simulink model "Passive_balancing"  (R2021b)
settings: Solver=VariableStepAuto  StartTime=0.0  StopTime=10.0  RelTol=1e-3
values from neighbouring files (symbols this model uses):
  I_cc = 4    [Passive_balancing.m]
  I_gain = 10    [Passive_balancing.m]
  P_gain = 100    [Passive_balancing.m]
  R_bleed = 20    [Passive_balancing.m]
  T_volt = 600    [Passive_balancing.m]
  V_top = 4.1    [Passive_balancing.m]
undefined symbols (not defined in the file or in its folder): Battery
libraries: fl_lib x36, nesl_utility x23, ee_lib x8, simulink x3, slpidlib x1
settings Model: Creator=vijay  LastModifiedBy=vijay

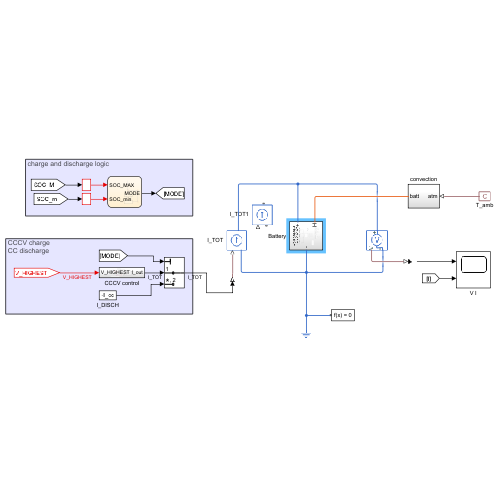
[thumbnail: Simulink's stored preview of the top-level diagram]
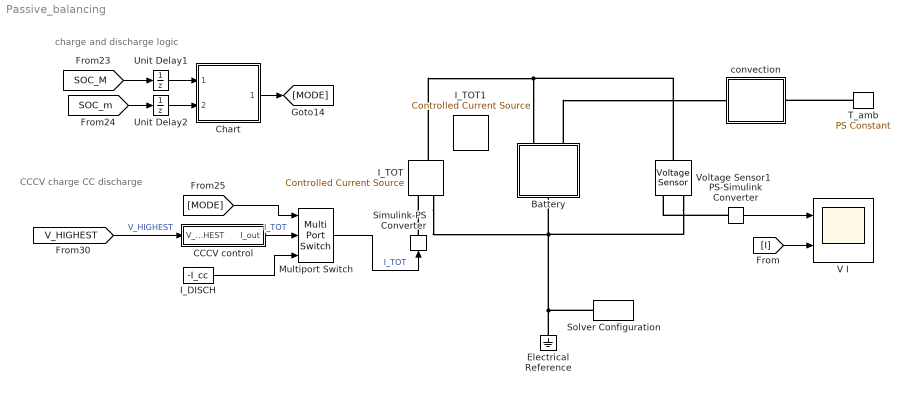
== system Passive_balancing ==
  note: charge and discharge logic
  note: CCCV charge
      | CC discharge
  Battery : Subsystem
  CCCV control : Subsystem
  Chart : Stateflow chart  TreatAsAtomicUnit=on
  Electrical Reference : fl_lib/Electrical/Electrical Elements/Electrical Reference
  I_DISCH : Constant  Value=-I_cc
  I_TOT : fl_lib/Electrical/Electrical Sources/Controlled Current Source
  I_TOT1 : fl_lib/Electrical/Electrical Sources/Controlled Current Source
  Multiport Switch : MultiPortSwitch  DataPortOrder=Specify indices  DataPortIndices={1,2}  DiagnosticForDefault=None
  PS-Simulink Converter : nesl_utility/PS-Simulink Converter  PhysicalDomain=network_engine_domain  SubClassName=ps_output  LeftPortType=input  RightPortType=output  PseudoPeriodic=off  Frequencies=[]  Unit=inherit  AffineConversion=off
      settings: SourceProductBaseCode=PW,SS
  Simulink-PS Converter : nesl_utility/Simulink-PS Converter  PhysicalDomain=network_engine_domain  SubClassName=ps_input  LeftPortType=input  RightPortType=output  PseudoPeriodic=off  Frequencies=[]  NoiseDistribution=none  NoiseParameters=[]  Unit=1  AffineConversion=off  FilteringAndDerivatives=provide  SimscapeFilterOrder=1  InputFilterTimeConstant=0.001  UdotUserProvided=0
      settings: SourceProductBaseCode=PW,SS
  Solver Configuration : nesl_utility/Solver Configuration  PhysicalDomain=network_engine_domain  SubClassName=solver  LeftPortType=input  RightPortType=generic  Tones=[]  Harmonics=[]  SimulateNoise=off  Profile=off  UseLocalSampling=off  EnableSwitchedLinearOptims=on  FrequencyDomain=off  UseCCode=off  RelTol=0.001  AbsTol=1e-06  MinStep=1e-09  ToWorkspace=off  RevertToSquareIcSolve=off  NumHomotopyIterations=100  PhasorMode=off  PhasorModeNumHarmonics=1  DoDC=off  ResidualTolerance=1e-09  UseLocalSolver=on  LocalSolverChoice=NE_BACKWARD_EULER_ADVANCER  LocalSolverSampleTime=1  DoFixedCost=on  MaxNonlinIter=3  MaxModeIter=2  ComputeImpulses=off  ImpulseIterations=2  LinearAlgebra=Sparse  EquationFormulation=NE_TIME_EF  DelaysMemoryBudget=1024  AutomaticFiltering=on  FilteringTimeConstant=0.001  PartitionStorageMethod=AS_NEEDED  PartitionMemoryBudget=1024  PartitionMethod=FAST
      settings: SourceProductBaseCode=PW,SS
  T_amb : fl_lib/Physical Signals/Sources/PS Constant  constant=20+273
  Unit Delay1 : UnitDelay  InitialCondition=1  SampleTime=-1  HasFrameUpgradeWarning=on
  Unit Delay2 : UnitDelay  InitialCondition=1  SampleTime=-1  HasFrameUpgradeWarning=on
  V I : Scope  NumInputPorts=2
  Voltage Sensor1 : fl_lib/Electrical/Electrical Sensors/Voltage Sensor
  convection : Subsystem
  wires:
  PS-Simulink Converter/1 -> V I/1
  [I] -> V I/2
  [V_HIGHEST] -> CCCV control/1(V_HIGHEST)  "V_HIGHEST"
  Unit Delay1/1 -> Chart/1(SOC_MAX)
  [SOC_M] -> Unit Delay1/1
  Unit Delay2/1 -> Chart/2(SOC_min)
  Chart/1(MODE) -> [MODE]
  I_DISCH/1 -> Multiport Switch/3
  CCCV control/1(I_out) -> Multiport Switch/2  "I_TOT"
  [SOC_m] -> Unit Delay2/1
  [MODE] -> Multiport Switch/1
  Multiport Switch/1 -> Simulink-PS Converter/1  "I_TOT"
  connections:
  Voltage Sensor1/LConn1 -- I_TOT/LConn1 -- Battery/LConn1
  Battery/LConn2 -- convection/LConn1
  Solver Configuration/RConn1 -- Voltage Sensor1/RConn2 -- I_TOT/RConn2 -- Battery/RConn1 -- Electrical Reference/LConn1
  T_amb/RConn1 -- convection/RConn1
  PS-Simulink Converter/LConn1 -- Voltage Sensor1/RConn1
  Simulink-PS Converter/RConn1 -- I_TOT/RConn1

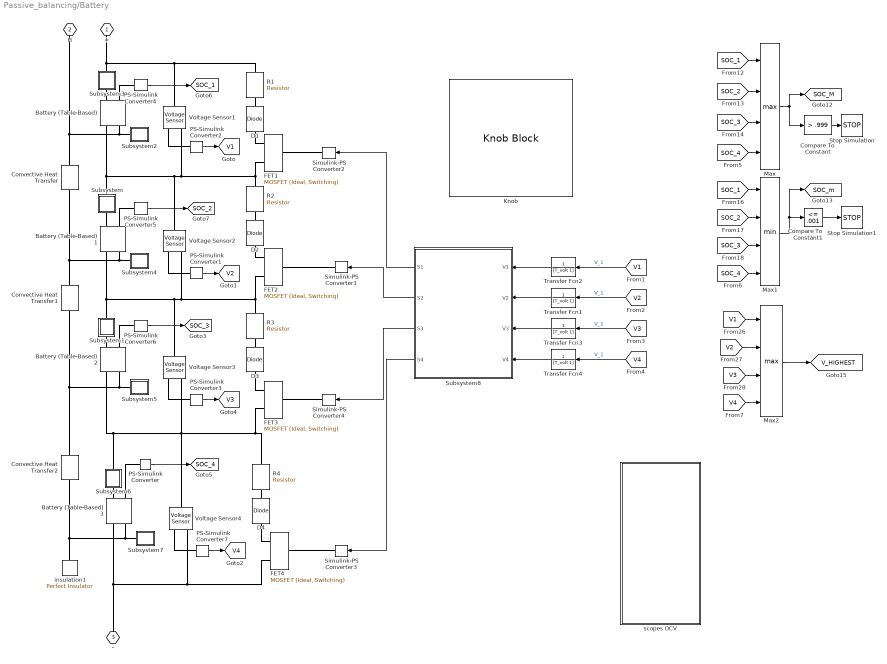
== system Passive_balancing/Battery ==
  Battery (Table-Based) : ee_lib/Sources/Battery (Table-Based)  SOC_vec=Battery(1).SOC_LUT  T_dependence=ee.enum.temperature_dependence.yes  prm_dir=ee.enum.battery.prm_dir.noCurrentDirectionality  T_vec=Battery(1).Temperature_LUT K  V0_mat=Battery(1).Em_LUT V  V0_vec=[3.1, 3.27, 3.31, 3.5] V  R0_mat=Battery(1).R0_LUT Ohm  R0_vec=[.015, .017, .012, .013] Ohm  R0_dis_mat=[.03, .015, .002; .04, .017, .008; .039, .012, .006; .027, .013, .021] Ohm  R0_dis_vec=[.015, .017, .012, .013] Ohm  R0_ch_mat=[.03, .015, .002; .04, .017, .008; .039, .012, .006; .027, .013, .021] Ohm  R0_ch_vec=[.015, .017, .012, .013] Ohm  AH_vec=Battery(1).Capacity_LUT A*hr  AH=4.1 A*hr  prm_leak=ee.enum.battery.prm_leak.disabled  Rleak_vec=[8000, 7000, 6000] Ohm  Rleak=7e3 Ohm  extrapolation_option=ee.enum.extrapolation.linear  prm_dyn=ee.enum.battery.prm_dyn.rc3  R1_mat=Battery(1).R1_LUT Ohm  R1_vec=[.076, .022, .007, .043] Ohm  tau1_mat=Battery(1).t1_LUT s  tau1_vec=[148, 110, 27, 22] s  R2_mat=Battery(1).R2_LUT Ohm  R2_vec=[.382, .006, .007, .956] Ohm  tau2_mat=Battery(1).t2_LUT s  tau2_vec=[44, 24, 14, 13419] s  R3_mat=Battery(1).R3_LUT Ohm  R3_vec=[.382, .006, .007, .956] Ohm  tau3_mat=Battery(1).t3_LUT s  tau3_vec=[44, 24, 14, 13419] s  R4_mat=Battery(1).R4_LUT Ohm  R4_vec=[.382, .006, .007, .956] Ohm  tau4_mat=Battery(1).t4_LUT s  tau4_vec=[44, 24, 14, 13419] s  R5_mat=[.014, .382, .407; .028, .006, .007; .014, .007, .006; .333, .956, .912] Ohm  R5_vec=[.382, .006, .007, .956] Ohm  tau5_mat=[1, 44, 5644; 11, 24, 506; 2, 14, 330; 3310, 13419, 30216] s  tau5_vec=[44, 24, 14, 13419] s  prm_fade=ee.enum.battery.prm_fade.equations  N0=100  dV0=0  dR0=0  dAH=0  dRleak=0  dR1=0  dR2=0  dR3=0  dR4=0  dR5=0  N0vec=[100, 200, 300]  Tfadevec=[298.15, 323.15] K  dV0vec=[0, 0, 0]  dR0vec=[0, 0, 0]  dAHvec=[0, 0, 0]  dRleakvec=[0, 0, 0]  dR1vec=[0, 0, 0]  dR2vec=[0, 0, 0]  dR3vec=[0, 0, 0]  dR4vec=[0, 0, 0]  dR5vec=[0, 0, 0]  dV0mat=[0, 0; 0, 0; 0, 0]  dR0mat=[0, 0; 0, 0; 0, 0]  dAHmat=[0, 0; 0, 0; 0, 0]  dRleakmat=[0, 0; 0, 0; 0, 0]  dR1mat=[0, 0; 0, 0; 0, 0]  dR2mat=[0, 0; 0, 0; 0, 0]  dR3mat=[0, 0; 0, 0; 0, 0]  dR4mat=[0, 0; 0, 0; 0, 0]  dR5mat=[0, 0; 0, 0; 0, 0]  prm_age=ee.enum.battery.prm_age.disabled  prm_age_OCV=ee.enum.battery.prm_age_OCV.OCV  OCV_age=0.9  SOC_age=0.6  storage_dt_age_vec=[0] d  storage_T_age_vec=[273] K  OCV_scaling_age=2.2134e6  OCV_offset_age=1.632e6  temp_exp_age=0.515833569 V  t_exp_age=0.75  T_age_vec=[273.15, 298.15, 323.15] K  dt_age_vec=[90, 180, 270, 360] d  dR0_age_vec=[0, 0, 0]  t_meas_dR0_age=100 d  dR0_age_mat=[0, 0, 0; 0, 0, 0; 0, 0, 0; 0, 0, 0]  temperature=Battery(1).T_init K  i_specify=off  i_priority=None  i=0 A  i_nominal_specify=off  i_nominal_unit=A  i_nominal_value=1  v_specify=off  v_priority=None  v=0 V  v_nominal_specify=off  v_nominal_unit=V  v_nominal_value=1  stateOfCharge_specify=on  stateOfCharge_priority=High  stateOfCharge=Battery(1).SOC0  stateOfCharge_nominal_specify=off  stateOfCharge_nominal_unit=1  stateOfCharge_nominal_value=1  num_cycles_specify=off  num_cycles_priority=High  num_cycles=0  num_cycles_nominal_specify=off  num_cycles_nominal_unit=1  num_cycles_nominal_value=1  thermal_mass=Battery(1).cell_Cp_heat * Battery(1).cell_mass J/K  temperature_specify=on  temperature_priority=High  temperature_nominal_specify=off  temperature_nominal_unit=K  temperature_nominal_value=1
      settings: SourceProductBaseCode=PS  InternalSimscapePortConfiguration="{\"Bottom\":[],\"Left\":[{\"id\":\"p\",\"label\":\"+\",\"type\":\"foundation.electrical.electrical\"},{\"id\":\"soc\",\"label\":\"SOC\",\"type\":\"output\"}],\"Right\":[{\"id\":\"n\",\"label\":\"-\",\"type\":\"foundation.electrical.electrical\"},{\"id\":\"H\",\"label\":\"H\",\"type\":\"foundation.thermal.thermal\"}],\"Top\":[]}"
  Battery (Table-Based)1 : ee_lib/Sources/Battery (Table-Based)  SOC_vec=Battery(2).SOC_LUT  T_dependence=ee.enum.temperature_dependence.yes  prm_dir=ee.enum.battery.prm_dir.noCurrentDirectionality  T_vec=Battery(2).Temperature_LUT K  V0_mat=Battery(2).Em_LUT V  V0_vec=[3.1, 3.27, 3.31, 3.5] V  R0_mat=Battery(2).R0_LUT Ohm  R0_vec=[.015, .017, .012, .013] Ohm  R0_dis_mat=[.03, .015, .002; .04, .017, .008; .039, .012, .006; .027, .013, .021] Ohm  R0_dis_vec=[.015, .017, .012, .013] Ohm  R0_ch_mat=[.03, .015, .002; .04, .017, .008; .039, .012, .006; .027, .013, .021] Ohm  R0_ch_vec=[.015, .017, .012, .013] Ohm  AH_vec=Battery(2).Capacity_LUT A*hr  AH=4.1 A*hr  prm_leak=ee.enum.battery.prm_leak.disabled  Rleak_vec=[8000, 7000, 6000] Ohm  Rleak=7e3 Ohm  extrapolation_option=ee.enum.extrapolation.linear  prm_dyn=ee.enum.battery.prm_dyn.rc3  R1_mat=Battery(2).R1_LUT Ohm  R1_vec=[.076, .022, .007, .043] Ohm  tau1_mat=Battery(2).t1_LUT s  tau1_vec=[148, 110, 27, 22] s  R2_mat=Battery(2).R2_LUT Ohm  R2_vec=[.382, .006, .007, .956] Ohm  tau2_mat=Battery(2).t2_LUT s  tau2_vec=[44, 24, 14, 13419] s  R3_mat=Battery(2).R3_LUT Ohm  R3_vec=[.382, .006, .007, .956] Ohm  tau3_mat=Battery(2).t3_LUT s  tau3_vec=[44, 24, 14, 13419] s  R4_mat=Battery(2).R4_LUT Ohm  R4_vec=[.382, .006, .007, .956] Ohm  tau4_mat=Battery(2).t4_LUT s  tau4_vec=[44, 24, 14, 13419] s  R5_mat=[.014, .382, .407; .028, .006, .007; .014, .007, .006; .333, .956, .912] Ohm  R5_vec=[.382, .006, .007, .956] Ohm  tau5_mat=[1, 44, 5644; 11, 24, 506; 2, 14, 330; 3310, 13419, 30216] s  tau5_vec=[44, 24, 14, 13419] s  prm_fade=ee.enum.battery.prm_fade.equations  N0=100  dV0=0  dR0=0  dAH=0  dRleak=0  dR1=0  dR2=0  dR3=0  dR4=0  dR5=0  N0vec=[100, 200, 300]  Tfadevec=[298.15, 323.15] K  dV0vec=[0, 0, 0]  dR0vec=[0, 0, 0]  dAHvec=[0, 0, 0]  dRleakvec=[0, 0, 0]  dR1vec=[0, 0, 0]  dR2vec=[0, 0, 0]  dR3vec=[0, 0, 0]  dR4vec=[0, 0, 0]  dR5vec=[0, 0, 0]  dV0mat=[0, 0; 0, 0; 0, 0]  dR0mat=[0, 0; 0, 0; 0, 0]  dAHmat=[0, 0; 0, 0; 0, 0]  dRleakmat=[0, 0; 0, 0; 0, 0]  dR1mat=[0, 0; 0, 0; 0, 0]  dR2mat=[0, 0; 0, 0; 0, 0]  dR3mat=[0, 0; 0, 0; 0, 0]  dR4mat=[0, 0; 0, 0; 0, 0]  dR5mat=[0, 0; 0, 0; 0, 0]  prm_age=ee.enum.battery.prm_age.disabled  prm_age_OCV=ee.enum.battery.prm_age_OCV.OCV  OCV_age=0.9  SOC_age=0.6  storage_dt_age_vec=[0] d  storage_T_age_vec=[273] K  OCV_scaling_age=2.2134e6  OCV_offset_age=1.632e6  temp_exp_age=0.515833569 V  t_exp_age=0.75  T_age_vec=[273.15, 298.15, 323.15] K  dt_age_vec=[90, 180, 270, 360] d  dR0_age_vec=[0, 0, 0]  t_meas_dR0_age=100 d  dR0_age_mat=[0, 0, 0; 0, 0, 0; 0, 0, 0; 0, 0, 0]  temperature=Battery(2).T_init K  i_specify=off  i_priority=None  i=0 A  i_nominal_specify=off  i_nominal_unit=A  i_nominal_value=1  v_specify=off  v_priority=None  v=0 V  v_nominal_specify=off  v_nominal_unit=V  v_nominal_value=1  stateOfCharge_specify=on  stateOfCharge_priority=High  stateOfCharge=Battery(2).SOC0  stateOfCharge_nominal_specify=off  stateOfCharge_nominal_unit=1  stateOfCharge_nominal_value=1  num_cycles_specify=off  num_cycles_priority=High  num_cycles=0  num_cycles_nominal_specify=off  num_cycles_nominal_unit=1  num_cycles_nominal_value=1  thermal_mass=Battery(2).cell_Cp_heat * Battery(2).cell_mass J/K  temperature_specify=on  temperature_priority=High  temperature_nominal_specify=off  temperature_nominal_unit=K  temperature_nominal_value=1
      settings: SourceProductBaseCode=PS  InternalSimscapePortConfiguration="{\"Bottom\":[],\"Left\":[{\"id\":\"p\",\"label\":\"+\",\"type\":\"foundation.electrical.electrical\"},{\"id\":\"soc\",\"label\":\"SOC\",\"type\":\"output\"}],\"Right\":[{\"id\":\"n\",\"label\":\"-\",\"type\":\"foundation.electrical.electrical\"},{\"id\":\"H\",\"label\":\"H\",\"type\":\"foundation.thermal.thermal\"}],\"Top\":[]}"
  Battery (Table-Based)2 : ee_lib/Sources/Battery (Table-Based)  SOC_vec=Battery(3).SOC_LUT  T_dependence=ee.enum.temperature_dependence.yes  prm_dir=ee.enum.battery.prm_dir.noCurrentDirectionality  T_vec=Battery(3).Temperature_LUT K  V0_mat=Battery(3).Em_LUT V  V0_vec=[3.1, 3.27, 3.31, 3.5] V  R0_mat=Battery(3).R0_LUT Ohm  R0_vec=[.015, .017, .012, .013] Ohm  R0_dis_mat=[.03, .015, .002; .04, .017, .008; .039, .012, .006; .027, .013, .021] Ohm  R0_dis_vec=[.015, .017, .012, .013] Ohm  R0_ch_mat=[.03, .015, .002; .04, .017, .008; .039, .012, .006; .027, .013, .021] Ohm  R0_ch_vec=[.015, .017, .012, .013] Ohm  AH_vec=Battery(3).Capacity_LUT A*hr  AH=4.1 A*hr  prm_leak=ee.enum.battery.prm_leak.disabled  Rleak_vec=[8000, 7000, 6000] Ohm  Rleak=7e3 Ohm  extrapolation_option=ee.enum.extrapolation.linear  prm_dyn=ee.enum.battery.prm_dyn.rc3  R1_mat=Battery(3).R1_LUT Ohm  R1_vec=[.076, .022, .007, .043] Ohm  tau1_mat=Battery(3).t1_LUT s  tau1_vec=[148, 110, 27, 22] s  R2_mat=Battery(3).R2_LUT Ohm  R2_vec=[.382, .006, .007, .956] Ohm  tau2_mat=Battery(3).t2_LUT s  tau2_vec=[44, 24, 14, 13419] s  R3_mat=Battery(3).R3_LUT Ohm  R3_vec=[.382, .006, .007, .956] Ohm  tau3_mat=Battery(3).t3_LUT s  tau3_vec=[44, 24, 14, 13419] s  R4_mat=Battery(3).R4_LUT Ohm  R4_vec=[.382, .006, .007, .956] Ohm  tau4_mat=Battery(3).t4_LUT s  tau4_vec=[44, 24, 14, 13419] s  R5_mat=[.014, .382, .407; .028, .006, .007; .014, .007, .006; .333, .956, .912] Ohm  R5_vec=[.382, .006, .007, .956] Ohm  tau5_mat=[1, 44, 5644; 11, 24, 506; 2, 14, 330; 3310, 13419, 30216] s  tau5_vec=[44, 24, 14, 13419] s  prm_fade=ee.enum.battery.prm_fade.equations  N0=100  dV0=0  dR0=0  dAH=0  dRleak=0  dR1=0  dR2=0  dR3=0  dR4=0  dR5=0  N0vec=[100, 200, 300]  Tfadevec=[298.15, 323.15] K  dV0vec=[0, 0, 0]  dR0vec=[0, 0, 0]  dAHvec=[0, 0, 0]  dRleakvec=[0, 0, 0]  dR1vec=[0, 0, 0]  dR2vec=[0, 0, 0]  dR3vec=[0, 0, 0]  dR4vec=[0, 0, 0]  dR5vec=[0, 0, 0]  dV0mat=[0, 0; 0, 0; 0, 0]  dR0mat=[0, 0; 0, 0; 0, 0]  dAHmat=[0, 0; 0, 0; 0, 0]  dRleakmat=[0, 0; 0, 0; 0, 0]  dR1mat=[0, 0; 0, 0; 0, 0]  dR2mat=[0, 0; 0, 0; 0, 0]  dR3mat=[0, 0; 0, 0; 0, 0]  dR4mat=[0, 0; 0, 0; 0, 0]  dR5mat=[0, 0; 0, 0; 0, 0]  prm_age=ee.enum.battery.prm_age.disabled  prm_age_OCV=ee.enum.battery.prm_age_OCV.OCV  OCV_age=0.9  SOC_age=0.6  storage_dt_age_vec=[0] d  storage_T_age_vec=[273] K  OCV_scaling_age=2.2134e6  OCV_offset_age=1.632e6  temp_exp_age=0.515833569 V  t_exp_age=0.75  T_age_vec=[273.15, 298.15, 323.15] K  dt_age_vec=[90, 180, 270, 360] d  dR0_age_vec=[0, 0, 0]  t_meas_dR0_age=100 d  dR0_age_mat=[0, 0, 0; 0, 0, 0; 0, 0, 0; 0, 0, 0]  temperature=Battery(3).T_init K  i_specify=off  i_priority=None  i=0 A  i_nominal_specify=off  i_nominal_unit=A  i_nominal_value=1  v_specify=off  v_priority=None  v=0 V  v_nominal_specify=off  v_nominal_unit=V  v_nominal_value=1  stateOfCharge_specify=on  stateOfCharge_priority=High  stateOfCharge=Battery(3).SOC0  stateOfCharge_nominal_specify=off  stateOfCharge_nominal_unit=1  stateOfCharge_nominal_value=1  num_cycles_specify=off  num_cycles_priority=High  num_cycles=0  num_cycles_nominal_specify=off  num_cycles_nominal_unit=1  num_cycles_nominal_value=1  thermal_mass=Battery(3).cell_Cp_heat * Battery(3).cell_mass J/K  temperature_specify=on  temperature_priority=High  temperature_nominal_specify=off  temperature_nominal_unit=K  temperature_nominal_value=1
      settings: SourceProductBaseCode=PS  InternalSimscapePortConfiguration="{\"Bottom\":[],\"Left\":[{\"id\":\"p\",\"label\":\"+\",\"type\":\"foundation.electrical.electrical\"},{\"id\":\"soc\",\"label\":\"SOC\",\"type\":\"output\"}],\"Right\":[{\"id\":\"n\",\"label\":\"-\",\"type\":\"foundation.electrical.electrical\"},{\"id\":\"H\",\"label\":\"H\",\"type\":\"foundation.thermal.thermal\"}],\"Top\":[]}"
  Battery (Table-Based)3 : ee_lib/Sources/Battery (Table-Based)  SOC_vec=Battery(3).SOC_LUT  T_dependence=ee.enum.temperature_dependence.yes  prm_dir=ee.enum.battery.prm_dir.noCurrentDirectionality  T_vec=Battery(3).Temperature_LUT K  V0_mat=Battery(3).Em_LUT V  V0_vec=[3.1, 3.27, 3.31, 3.5] V  R0_mat=Battery(3).R0_LUT Ohm  R0_vec=[.015, .017, .012, .013] Ohm  R0_dis_mat=[.03, .015, .002; .04, .017, .008; .039, .012, .006; .027, .013, .021] Ohm  R0_dis_vec=[.015, .017, .012, .013] Ohm  R0_ch_mat=[.03, .015, .002; .04, .017, .008; .039, .012, .006; .027, .013, .021] Ohm  R0_ch_vec=[.015, .017, .012, .013] Ohm  AH_vec=Battery(3).Capacity_LUT A*hr  AH=4.1 A*hr  prm_leak=ee.enum.battery.prm_leak.disabled  Rleak_vec=[8000, 7000, 6000] Ohm  Rleak=7e3 Ohm  extrapolation_option=ee.enum.extrapolation.linear  prm_dyn=ee.enum.battery.prm_dyn.rc3  R1_mat=Battery(3).R1_LUT Ohm  R1_vec=[.076, .022, .007, .043] Ohm  tau1_mat=Battery(3).t1_LUT s  tau1_vec=[148, 110, 27, 22] s  R2_mat=Battery(3).R2_LUT Ohm  R2_vec=[.382, .006, .007, .956] Ohm  tau2_mat=Battery(3).t2_LUT s  tau2_vec=[44, 24, 14, 13419] s  R3_mat=Battery(3).R3_LUT Ohm  R3_vec=[.382, .006, .007, .956] Ohm  tau3_mat=Battery(3).t3_LUT s  tau3_vec=[44, 24, 14, 13419] s  R4_mat=Battery(3).R4_LUT Ohm  R4_vec=[.382, .006, .007, .956] Ohm  tau4_mat=Battery(3).t4_LUT s  tau4_vec=[44, 24, 14, 13419] s  R5_mat=[.014, .382, .407; .028, .006, .007; .014, .007, .006; .333, .956, .912] Ohm  R5_vec=[.382, .006, .007, .956] Ohm  tau5_mat=[1, 44, 5644; 11, 24, 506; 2, 14, 330; 3310, 13419, 30216] s  tau5_vec=[44, 24, 14, 13419] s  prm_fade=ee.enum.battery.prm_fade.equations  N0=100  dV0=0  dR0=0  dAH=0  dRleak=0  dR1=0  dR2=0  dR3=0  dR4=0  dR5=0  N0vec=[100, 200, 300]  Tfadevec=[298.15, 323.15] K  dV0vec=[0, 0, 0]  dR0vec=[0, 0, 0]  dAHvec=[0, 0, 0]  dRleakvec=[0, 0, 0]  dR1vec=[0, 0, 0]  dR2vec=[0, 0, 0]  dR3vec=[0, 0, 0]  dR4vec=[0, 0, 0]  dR5vec=[0, 0, 0]  dV0mat=[0, 0; 0, 0; 0, 0]  dR0mat=[0, 0; 0, 0; 0, 0]  dAHmat=[0, 0; 0, 0; 0, 0]  dRleakmat=[0, 0; 0, 0; 0, 0]  dR1mat=[0, 0; 0, 0; 0, 0]  dR2mat=[0, 0; 0, 0; 0, 0]  dR3mat=[0, 0; 0, 0; 0, 0]  dR4mat=[0, 0; 0, 0; 0, 0]  dR5mat=[0, 0; 0, 0; 0, 0]  prm_age=ee.enum.battery.prm_age.disabled  prm_age_OCV=ee.enum.battery.prm_age_OCV.OCV  OCV_age=0.9  SOC_age=0.6  storage_dt_age_vec=[0] d  storage_T_age_vec=[273] K  OCV_scaling_age=2.2134e6  OCV_offset_age=1.632e6  temp_exp_age=0.515833569 V  t_exp_age=0.75  T_age_vec=[273.15, 298.15, 323.15] K  dt_age_vec=[90, 180, 270, 360] d  dR0_age_vec=[0, 0, 0]  t_meas_dR0_age=100 d  dR0_age_mat=[0, 0, 0; 0, 0, 0; 0, 0, 0; 0, 0, 0]  temperature=Battery(3).T_init K  i_specify=off  i_priority=None  i=0 A  i_nominal_specify=off  i_nominal_unit=A  i_nominal_value=1  v_specify=off  v_priority=None  v=0 V  v_nominal_specify=off  v_nominal_unit=V  v_nominal_value=1  stateOfCharge_specify=on  stateOfCharge_priority=High  stateOfCharge=Battery(3).SOC0  stateOfCharge_nominal_specify=off  stateOfCharge_nominal_unit=1  stateOfCharge_nominal_value=1  num_cycles_specify=off  num_cycles_priority=High  num_cycles=0  num_cycles_nominal_specify=off  num_cycles_nominal_unit=1  num_cycles_nominal_value=1  thermal_mass=Battery(3).cell_Cp_heat * Battery(3).cell_mass J/K  temperature_specify=on  temperature_priority=High  temperature_nominal_specify=off  temperature_nominal_unit=K  temperature_nominal_value=1
      settings: SourceProductBaseCode=PS  InternalSimscapePortConfiguration="{\"Bottom\":[],\"Left\":[{\"id\":\"p\",\"label\":\"+\",\"type\":\"foundation.electrical.electrical\"},{\"id\":\"soc\",\"label\":\"SOC\",\"type\":\"output\"}],\"Right\":[{\"id\":\"n\",\"label\":\"-\",\"type\":\"foundation.electrical.electrical\"},{\"id\":\"H\",\"label\":\"H\",\"type\":\"foundation.thermal.thermal\"}],\"Top\":[]}"
  Compare To Constant : simulink/Logic and Bit Operations/Compare To Constant  relop=>  const=.999  OutDataTypeStr=boolean
  Compare To Constant1 : simulink/Logic and Bit Operations/Compare To Constant  relop=<=  const=.001  OutDataTypeStr=boolean
  Convective Heat Transfer : fl_lib/Thermal/Thermal Elements/Convective Heat Transfer  area=cell_area m^2  heat_tr_coeff=h_conv W/(m^2 * K)  T_specify=off  T_priority=None  T=0 K  T_nominal_specify=off  T_nominal_unit=K  T_nominal_value=1  Q_specify=off  Q_priority=None  Q=0 J/s  Q_nominal_specify=off  Q_nominal_unit=J/s  Q_nominal_value=1
  Convective Heat Transfer1 : fl_lib/Thermal/Thermal Elements/Convective Heat Transfer  area=cell_area m^2  heat_tr_coeff=h_conv W/(m^2 * K)  T_specify=off  T_priority=None  T=0 K  T_nominal_specify=off  T_nominal_unit=K  T_nominal_value=1  Q_specify=off  Q_priority=None  Q=0 J/s  Q_nominal_specify=off  Q_nominal_unit=J/s  Q_nominal_value=1
  Convective Heat Transfer2 : fl_lib/Thermal/Thermal Elements/Convective Heat Transfer  area=cell_area m^2  heat_tr_coeff=h_conv W/(m^2 * K)  T_specify=off  T_priority=None  T=0 K  T_nominal_specify=off  T_nominal_unit=K  T_nominal_value=1  Q_specify=off  Q_priority=None  Q=0 J/s  Q_nominal_specify=off  Q_nominal_unit=J/s  Q_nominal_value=1
  D{1..4} (4 alike) : fl_lib/Electrical/Electrical Elements/Diode  Vf=0.6 V  Ron=0.3 Ohm  Goff=1e-8 1/Ohm  i_specify=off  i_priority=None  i=0 A  i_nominal_specify=off  i_nominal_unit=A  i_nominal_value=1  v_specify=off  v_priority=None  v=0 V  v_nominal_specify=off  v_nominal_unit=V  v_nominal_value=1
      settings: LogSimulationData=on
  FET{1..4} (4 alike) : ee_lib/Semiconductors & Converters/MOSFET (Ideal, Switching)  Rds=0.01 Ohm  Goff=1e-6 1/Ohm  Vth=0.9 V  diode_param=2  diode_Vf=0.8 V  diode_Ron=0.001 Ohm  diode_Goff=1e-5 1/Ohm  diode_C=5e-8 F  diode_iRM=-235 A  diode_iF=300 A  diode_idot=-50 A/us  diode_trr_param=1  diode_trr_factor=3  diode_trr=15 us  diode_Qrr=1.5e+3 s*uA  thermal_loss_option=ee.enum.converters.thermalLossOption.constantvalues  Von_data=[0, 1.1, 1.3, 1.45, 1.75, 2.25, 2.7; 0, 1, 1.15, 1.35, 1.7, 2.35, 3] V  Tj=[298.15, 398.15] K  Iout_data=[0, 10, 50, 100, 200, 400, 600] A  Eon_data=[0, .29, 1.43, 2.86, 5.71, 13.14, 22.86; 0, .57, 2.63, 5.14, 10.29, 20.57, 30.29] * 1e-3 J  Eoff_data=[0, .21, 1.07, 2.14, 4.29, 9.86, 17.14; 0, .43, 1.97, 3.86, 7.71, 15.43, 22.71] * 1e-3 J  Tj_loss=[298.15, 398.15] K  Iout_data_loss=[0, 10, 50, 100, 200, 400, 600] A  Eon_scalar=22.86e-3 J  Eoff_scalar=17.14e-3 J  Voff=300 V  Iout_scalar=600 A  diodeModelType=ee.enum.converters.diodeModelType.pwl  diodeTableType=ee.enum.diode.tableType.IfMat  diode_IfMat=[.07, .12, .19, 1.75, 4.24, 7.32, 11.2; .16, .3, .72, 2.14, 4.02, 6.35, 9.12] A  diode_VfMat=[.9, 1.15, 1.25, 1.5, 1.75, 2.17, 2.6, 2.85; .58, .68, .75, 1.1, 1.38, 1.77, 2.27, 2.7] V  diode_TjVec=[25, 125] degC  diode_VfVec=[.5, .7, .9, 1.3, 1.7, 2.1, 2.5] V  diode_IfVec=[.1, .2, .5, 1, 2, 4, 7, 10] A  diode_Vr=-600 V  diode_Ls=150 nH  diode_Erec=0.03 J  thermal_network_parameterization=ee.enum.thermalNetworkTopology.external  Rth=[.03, .2] K/W  Rth_Cauer=[.03, .1, .2] K/W  Rth_Foster=[.03, .2] K/W  thermal_mass_parameterization=ee.enum.thermalNetwork.timeconstant  thermal_mass=[3, 25] J/K  thermal_mass_Cauer=[3, 10, 25] J/K  thermal_mass_Foster=[33, 50] J/K  thermal_time_constant=[.1, 5] s  thermal_time_constant_Cauer=[.1, 1, 5] s  thermal_time_constant_Foster=[1, 10] s  thermal_mass_initial_temperatures=[25, 25] degC  thermal_mass_initial_temperatures_Cauer=[25, 25, 25] degC  junction_thermal_mass=0.1 J/K  steadyState_Foster=simscape.enum.onoff.on  Tvec_initial_Foster=[25, 25, 25, 25] degC  no_thermal_network=0  junction_temperature_specify=off  junction_temperature_priority=None  junction_temperature=25 degC  junction_temperature_nominal_specify=off  junction_temperature_nominal_unit=degC  junction_temperature_nominal_value=1  vT_specify=off  vT_priority=None  vT=0 V  vT_nominal_specify=off  vT_nominal_unit=V  vT_nominal_value=1  Qj_specify=off  Qj_priority=None  Qj=0 W  Qj_nominal_specify=off  Qj_nominal_unit=W  Qj_nominal_value=1
  Knob : KnobBlock  ScaleMin=2  ScaleMax=40
  Max : MinMax  Function=max  Inputs=4
  Max1 : MinMax  Inputs=4
  Max2 : MinMax  Function=max  Inputs=4
  PS-Simulink Converter : nesl_utility/PS-Simulink Converter  PhysicalDomain=network_engine_domain  SubClassName=ps_output  LeftPortType=input  RightPortType=output  PseudoPeriodic=off  Frequencies=[]  Unit=inherit  AffineConversion=off
      settings: SourceProductBaseCode=PW,SS
  PS-Simulink Converter{1..7} (7 alike) : nesl_utility/PS-Simulink Converter  PhysicalDomain=network_engine_domain  SubClassName=ps_output  LeftPortType=input  RightPortType=output  PseudoPeriodic=off  Frequencies=[]  Unit=1  AffineConversion=off
  R{1..4} (4 alike) : fl_lib/Electrical/Electrical Elements/Resistor  R=R_bleed Ohm  i_specify=off  i_priority=None  i=0 A  i_nominal_specify=off  i_nominal_unit=A  i_nominal_value=1  v_specify=off  v_priority=None  v=0 V  v_nominal_specify=off  v_nominal_unit=V  v_nominal_value=1
      R1 settings: LogSimulationData=on
  Simulink-PS Converter{1..4} (4 alike) : nesl_utility/Simulink-PS Converter  PhysicalDomain=network_engine_domain  SubClassName=ps_input  LeftPortType=input  RightPortType=output  PseudoPeriodic=off  Frequencies=[]  NoiseDistribution=none  NoiseParameters=[]  Unit=1  AffineConversion=off  FilteringAndDerivatives=zero  SimscapeFilterOrder=1  InputFilterTimeConstant=0.001  UdotUserProvided=1
  Stop Simulation : Stop
  Stop Simulation1 : Stop
  Subsystem : Subsystem
  Subsystem1 : Subsystem
  Subsystem2 : Subsystem
  Subsystem3 : Subsystem
  Subsystem4 : Subsystem
  Subsystem5 : Subsystem
  Subsystem6 : Subsystem
  Subsystem7 : Subsystem
  Subsystem8 : Subsystem
  Transfer Fcn{1..4} (4 alike) : TransferFcn  Denominator=[T_volt 1]
  Voltage Sensor{1..4} (4 alike) : fl_lib/Electrical/Electrical Sensors/Voltage Sensor
  insulation1 : fl_lib/Thermal/Thermal Elements/Perfect Insulator  T_specify=off  T_priority=None  T=0 K  T_nominal_specify=off  T_nominal_unit=K  T_nominal_value=1
  scopes OCV : Subsystem
  + : PMIOPort  Side=Left
  H : PMIOPort  Port=2  Side=Left
  - : PMIOPort  Port=3  Side=Right
  tag scope: SOC_1=global, SOC_2=global, SOC_3=global, SOC_4=global, SOC_M=global, SOC_m=global, V1=global, V2=global, V3=global, V4=global, V_HIGHEST=global
  wires:
  Compare To Constant1/1 -> Stop Simulation1/1
  Transfer Fcn4/1 -> Subsystem8/4(V4)
  PS-Simulink Converter7/1 -> [V4]
  Max/1 -> Compare To Constant/1, [SOC_M]
  [SOC_3] -> Max1/3
  [V2] -> Max2/2
  PS-Simulink Converter3/1 -> [V3]
  [V3] -> Max2/3
  [V1] -> Transfer Fcn2/1  "V_1"
  [SOC_2] -> Max/2
  PS-Simulink Converter5/1 -> [SOC_2]
  PS-Simulink Converter/1 -> [SOC_4]
  Subsystem8/2(S2) -> Simulink-PS Converter1/1
  Transfer Fcn1/1 -> Subsystem8/2(V2)
  [V4] -> Transfer Fcn4/1  "V_1"
  Transfer Fcn3/1 -> Subsystem8/3(V3)
  Subsystem8/4(S4) -> Simulink-PS Converter3/1
  Subsystem8/3(S3) -> Simulink-PS Converter4/1
  Transfer Fcn2/1 -> Subsystem8/1(V1)
  Max1/1 -> Compare To Constant1/1, [SOC_m]
  [V2] -> Transfer Fcn1/1  "V_1"
  [V3] -> Transfer Fcn3/1  "V_1"
  [SOC_2] -> Max1/2
  [V4] -> Max2/4
  PS-Simulink Converter4/1 -> [SOC_1]
  PS-Simulink Converter6/1 -> [SOC_3]
  PS-Simulink Converter2/1 -> [V1]
  [SOC_4] -> Max/4
  PS-Simulink Converter1/1 -> [V2]
  Subsystem8/1(S1) -> Simulink-PS Converter2/1
  [SOC_4] -> Max1/4
  [SOC_1] -> Max/1
  Max2/1 -> [V_HIGHEST]
  [V1] -> Max2/1
  [SOC_3] -> Max/3
  Compare To Constant/1 -> Stop Simulation/1
  [SOC_1] -> Max1/1
  connections:
  R2/LConn1 -- FET1/RConn2 -- Subsystem/LConn1 -- Battery (Table-Based)/RConn1 -- Voltage Sensor2/LConn1 -- Voltage Sensor1/RConn2
  Convective Heat Transfer1/LConn1 -- Convective Heat Transfer/RConn1 -- Subsystem4/LConn1 -- Battery (Table-Based)1/RConn2
  Battery (Table-Based)3/LConn2 -- PS-Simulink Converter/LConn1
  Simulink-PS Converter3/RConn1 -- FET4/LConn1
  PS-Simulink Converter3/LConn1 -- Voltage Sensor3/RConn1
  Voltage Sensor3/RConn2 -- R4/LConn1 -- FET3/RConn2 -- Voltage Sensor4/LConn1 -- Battery (Table-Based)2/RConn1 -- Subsystem6/LConn1
  Simulink-PS Converter1/RConn1 -- FET2/LConn1
  FET4/RConn1 -- D4/RConn1
  Voltage Sensor4/RConn2 -- -/RConn1 -- Battery (Table-Based)3/RConn1 -- FET4/RConn2
  R4/RConn1 -- D4/LConn1
  R3/LConn1 -- FET2/RConn2 -- Voltage Sensor2/RConn2 -- Battery (Table-Based)1/RConn1 -- Subsystem1/LConn1 -- Voltage Sensor3/LConn1
  Battery (Table-Based)/LConn1 -- Subsystem3/RConn1
  Battery (Table-Based)3/LConn1 -- Subsystem6/RConn1
  insulation1/LConn1 -- Battery (Table-Based)3/RConn2 -- Subsystem7/LConn1 -- Convective Heat Transfer2/RConn1
  FET1/RConn1 -- D1/RConn1
  PS-Simulink Converter7/LConn1 -- Voltage Sensor4/RConn1
  Subsystem3/LConn1 -- +/RConn1 -- Voltage Sensor1/LConn1 -- R1/LConn1
  PS-Simulink Converter1/LConn1 -- Voltage Sensor2/RConn1
  Simulink-PS Converter2/RConn1 -- FET1/LConn1
  Battery (Table-Based)2/LConn1 -- Subsystem1/RConn1
  FET3/RConn1 -- D3/RConn1
  Battery (Table-Based)/RConn2 -- Subsystem2/LConn1 -- H/RConn1 -- Convective Heat Transfer/LConn1
  Subsystem5/LConn1 -- Battery (Table-Based)2/RConn2 -- Convective Heat Transfer2/LConn1 -- Convective Heat Transfer1/RConn1
  Battery (Table-Based)2/LConn2 -- PS-Simulink Converter6/LConn1
  Battery (Table-Based)1/LConn1 -- Subsystem/RConn1
  R2/RConn1 -- D2/LConn1
  Battery (Table-Based)/LConn2 -- PS-Simulink Converter4/LConn1
  PS-Simulink Converter2/LConn1 -- Voltage Sensor1/RConn1
  R3/RConn1 -- D3/LConn1
  Battery (Table-Based)1/LConn2 -- PS-Simulink Converter5/LConn1
  R1/RConn1 -- D1/LConn1
  FET2/RConn1 -- D2/RConn1
  Simulink-PS Converter4/RConn1 -- FET3/LConn1

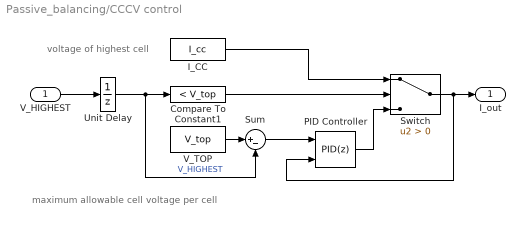
== system Passive_balancing/CCCV control ==
  note: maximum allowable cell voltage per cell
  note: voltage of highest cell
  V_HIGHEST : Inport
  Compare To Constant1 : simulink/Logic and Bit Operations/Compare To Constant  relop=<  const=V_top  OutDataTypeStr=boolean
  I_CC : Constant  Value=I_cc
  PID Controller : slpidlib/PID Controller  Controller=PID  Form=Parallel  TimeDomain=Discrete-time  UseExternalTs=off  SampleTime=1  IntegratorMethod=Forward Euler  FilterMethod=Forward Euler  ControllerParametersSource=internal  P=P_gain  I=I_gain  D=0  UseFilter=on  N=100  TunerSelectOption=Transfer Function Based (PID Tuner App)  InitialConditionSource=internal  InitialConditionForIntegrator=10  InitialConditionForFilter=0  DifferentiatorICPrevScaledInput=0  ExternalReset=none  TrackingMode=on  Kt=1  LimitOutput=on  SatLimitsSource=internal  UpperSaturationLimit=Inf  LowerSaturationLimit=0  LinearizeAsGain=on  AntiWindupMode=clamping  Kb=1  POutMin=[]  POutMax=[]  IOutMin=[]  IOutMax=[]  DOutMin=[]  DOutMax=[]  NOutMin=[]  NOutMax=[]  SumOutMin=[]  SumOutMax=[]  SaturationOutMin=[]  SaturationOutMax=[]  PParamMin=[]  PParamMax=[]  IParamMin=[]  IParamMax=[]  DParamMin=[]  DParamMax=[]  NParamMin=[]  NParamMax=[]  KbParamMin=[]  KbParamMax=[]  KtParamMin=[]  KtParamMax=[]  KbOutMin=[]  KbOutMax=[]  KtOutMin=[]  KtOutMax=[]  IntegratorOutMin=[]  IntegratorOutMax=[]  FilterOutMin=[]  FilterOutMax=[]  SumI1OutMin=[]  SumI1OutMax=[]  SumI2OutMin=[]  SumI2OutMax=[]  SumI3OutMin=[]  SumI3OutMax=[]  SumI4OutMin=[]  SumI4OutMax=[]  SumDOutMin=[]  SumDOutMax=[]  DifferentiatorOutMin=[]  DifferentiatorOutMax=[]  FilterDiffOutCoefMin=[]  FilterDiffOutCoefMax=[]  ReciprocalOutMin=[]  ReciprocalOutMax=[]  SumDenOutMin=[]  SumDenOutMax=[]  SumNumOutMin=[]  SumNumOutMax=[]  DivideOutMin=[]  DivideOutMax=[]  UdiffTsProdOutMin=[]  UdiffTsProdOutMax=[]  NTsProdOutMin=[]  NTsProdOutMax=[]  UintegralTsProdOutMin=[]  UintegralTsProdOutMax=[]  UngainTsProdOutMin=[]  UngainTsProdOutMax=[]  IntegratorContinuousStateAttributes=''  IntegratorStateMustResolveToSignalObject=off  IntegratorRTWStateStorageClass=Auto  FilterContinuousStateAttributes=''  FilterStateMustResolveToSignalObject=off  FilterRTWStateStorageClass=Auto  ParallelPVariant=InternalParameters  IdealPVariant=Disabled  IVariant=InternalParameters  DVariant=InternalParameters  IntegratorVariant=Discrete  SatVariant=Enabled  AWVariant=DiscClampingParallel  PCopyVariant=Disabled  TRVariant=Enabled  FdbkBlocksVariant=Forward  IdealPFdbkVariant=Disabled  SatFdbkVariant=Disabled  DerivativeFilterVariant=ForwardEulerFilter  NVariant=InternalParameters  NCopyVariant=Disabled  FilterICVariant=InternalICsFilter  IntegratorICVariant=InternalICs  ExternalResetVariant=Disabled  TRSumVariant=TrackingMode  SumFdbkVariant=Disabled  SumVariant=Sum_PID  TsampFilterVariant=InternalTs  TsampNgainVariant=Passthrough  TsampIntegralVariant=Passthrough  ExternalSaturationOutDataTypeStr=Inherit: Same as second input
  Sum : Sum  Inputs=|+-
  Switch : Switch  Criteria=u2 > Threshold
  Unit Delay : UnitDelay  SampleTime=-1  HasFrameUpgradeWarning=on
  V_TOP : Constant  Value=V_top
  I_out : Outport
  wires:
  Switch/1 -> I_out/1, PID Controller/2
  Unit Delay/1 -> Sum/2, Compare To Constant1/1  "V_HIGHEST"
  PID Controller/1 -> Switch/3
  Sum/1 -> PID Controller/1
  V_TOP/1 -> Sum/1
  I_CC/1 -> Switch/1
  V_HIGHEST/1 -> Unit Delay/1
  Compare To Constant1/1 -> Switch/2

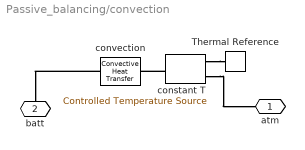
== system Passive_balancing/convection ==
  Thermal Reference : fl_lib/Thermal/Thermal Elements/Thermal Reference
  constant T : fl_lib/Thermal/Thermal Sources/Controlled Temperature Source
  convection : fl_lib/Thermal/Thermal Elements/Convective Heat Transfer  area=cell_area m^2  heat_tr_coeff=h_conv W/(m^2 * K)  T_specify=off  T_priority=None  T=0 K  T_nominal_specify=off  T_nominal_unit=K  T_nominal_value=1  Q_specify=off  Q_priority=None  Q=0 J/s  Q_nominal_specify=off  Q_nominal_unit=J/s  Q_nominal_value=1
  atm : PMIOPort  Side=Right
  batt : PMIOPort  Port=2  Side=Left
  connections:
  convection/LConn1 -- batt/RConn1
  constant T/LConn1 -- convection/RConn1
  constant T/RConn2 -- Thermal Reference/LConn1
  constant T/RConn1 -- atm/RConn1

== system Passive_balancing/Battery/Subsystem ==
  Subsystem1 : Subsystem
  1 : PMIOPort  Side=Left
  2 : PMIOPort  Port=2  Side=Right
  tag scope: I2=global
  wires:
  Subsystem1/1(3) -> [I2]
  connections:
  Subsystem1/LConn1 -- 1/RConn1
  Subsystem1/RConn1 -- 2/RConn1

== system Passive_balancing/Battery/Subsystem1 ==
  Subsystem2 : Subsystem
  1 : PMIOPort  Side=Left
  2 : PMIOPort  Port=2  Side=Right
  tag scope: I3=global
  wires:
  Subsystem2/1(3) -> [I3]
  connections:
  Subsystem2/RConn1 -- 2/RConn1
  Subsystem2/LConn1 -- 1/RConn1

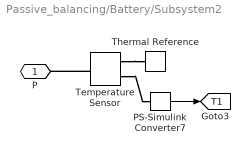
== system Passive_balancing/Battery/Subsystem2 ==
  PS-Simulink Converter7 : nesl_utility/PS-Simulink Converter  PhysicalDomain=network_engine_domain  SubClassName=ps_output  LeftPortType=input  RightPortType=output  PseudoPeriodic=off  Frequencies=[]  Unit=degC  AffineConversion=on
  Temperature Sensor : fl_lib/Thermal/Thermal Sensors/Temperature Sensor
  Thermal Reference : fl_lib/Thermal/Thermal Elements/Thermal Reference
  P : PMIOPort  Side=Left
  tag scope: T1=global
  wires:
  PS-Simulink Converter7/1 -> [T1]
  connections:
  Temperature Sensor/RConn1 -- Thermal Reference/LConn1
  Temperature Sensor/LConn1 -- P/RConn1
  Temperature Sensor/RConn2 -- PS-Simulink Converter7/LConn1

== system Passive_balancing/Battery/Subsystem3 ==
  Subsystem : Subsystem
  1 : PMIOPort  Side=Left
  2 : PMIOPort  Port=2  Side=Right
  tag scope: I1=global
  wires:
  Subsystem/1(3) -> [I1]
  connections:
  Subsystem/RConn1 -- 2/RConn1
  Subsystem/LConn1 -- 1/RConn1

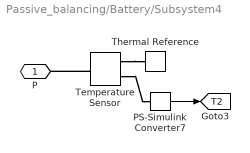
== system Passive_balancing/Battery/Subsystem4 ==
  PS-Simulink Converter7 : nesl_utility/PS-Simulink Converter  PhysicalDomain=network_engine_domain  SubClassName=ps_output  LeftPortType=input  RightPortType=output  PseudoPeriodic=off  Frequencies=[]  Unit=degC  AffineConversion=on
  Temperature Sensor : fl_lib/Thermal/Thermal Sensors/Temperature Sensor
  Thermal Reference : fl_lib/Thermal/Thermal Elements/Thermal Reference
  P : PMIOPort  Side=Left
  tag scope: T2=global
  wires:
  PS-Simulink Converter7/1 -> [T2]
  connections:
  Temperature Sensor/RConn2 -- PS-Simulink Converter7/LConn1
  Temperature Sensor/LConn1 -- P/RConn1
  Temperature Sensor/RConn1 -- Thermal Reference/LConn1

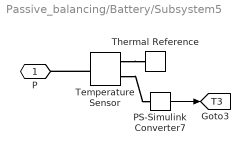
== system Passive_balancing/Battery/Subsystem5 ==
  PS-Simulink Converter7 : nesl_utility/PS-Simulink Converter  PhysicalDomain=network_engine_domain  SubClassName=ps_output  LeftPortType=input  RightPortType=output  PseudoPeriodic=off  Frequencies=[]  Unit=degC  AffineConversion=on
  Temperature Sensor : fl_lib/Thermal/Thermal Sensors/Temperature Sensor
  Thermal Reference : fl_lib/Thermal/Thermal Elements/Thermal Reference
  P : PMIOPort  Side=Left
  tag scope: T3=global
  wires:
  PS-Simulink Converter7/1 -> [T3]
  connections:
  Temperature Sensor/RConn1 -- Thermal Reference/LConn1
  Temperature Sensor/LConn1 -- P/RConn1
  Temperature Sensor/RConn2 -- PS-Simulink Converter7/LConn1

== system Passive_balancing/Battery/Subsystem6 ==
  Subsystem2 : Subsystem
  1 : PMIOPort  Side=Left
  2 : PMIOPort  Port=2  Side=Right
  tag scope: I4=global
  wires:
  Subsystem2/1(3) -> [I4]
  connections:
  Subsystem2/RConn1 -- 2/RConn1
  Subsystem2/LConn1 -- 1/RConn1

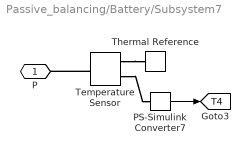
== system Passive_balancing/Battery/Subsystem7 ==
  PS-Simulink Converter7 : nesl_utility/PS-Simulink Converter  PhysicalDomain=network_engine_domain  SubClassName=ps_output  LeftPortType=input  RightPortType=output  PseudoPeriodic=off  Frequencies=[]  Unit=degC  AffineConversion=on
  Temperature Sensor : fl_lib/Thermal/Thermal Sensors/Temperature Sensor
  Thermal Reference : fl_lib/Thermal/Thermal Elements/Thermal Reference
  P : PMIOPort  Side=Left
  tag scope: T4=global
  wires:
  PS-Simulink Converter7/1 -> [T4]
  connections:
  Temperature Sensor/RConn1 -- Thermal Reference/LConn1
  Temperature Sensor/LConn1 -- P/RConn1
  Temperature Sensor/RConn2 -- PS-Simulink Converter7/LConn1

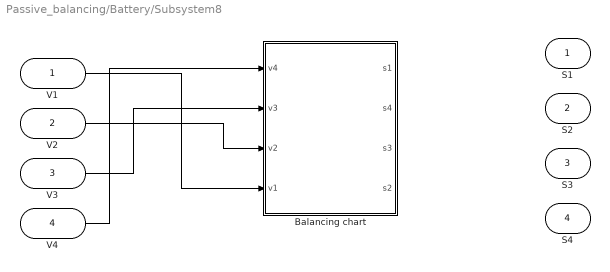
== system Passive_balancing/Battery/Subsystem8 ==
  V1 : Inport
  V2 : Inport  Port=2
  V3 : Inport  Port=3
  V4 : Inport  Port=4
  Balancing chart : Stateflow chart  TreatAsAtomicUnit=on
      settings: PortSchema="{\"entries\":[{\"content\":{\"sides\":[{\"content\":{\"connectorIds\":[\"In1\",\"In3\",\"In2\",\"In4\"]},\"type\":\"ConnectorPlacement.EquallySpacedRectSide\",\"uuid\":\"59b0e5e9-bda9-4177-8cf3-a454171fc9b7\"},{\"content\":{\"connectorIds\":[\"Out1\",\"Out2\",\"Out3\",\"Out4\"],\"side\":\"RIGHT\"},\"type\":\"ConnectorPlacement.EquallySpacedRectSide\",\"uuid\":\"9fbfc770-3965-4493-b4fe-4e1e12ae5365\"},{\"content\":{\"connectorIds\":[],\"side\":\"TOP\"},\"type\":\"ConnectorPlacement.EquallySpacedRectSide\",\"uuid\":\"18bbd589-0de7-4df3-912a-6991e421f4e8\"}]},\"type\":\"ConnectorPlacement.EquallySpacedConnector\",\"uuid\":\"dd5c23fc-6f73-40d1-893b-db7cae84196b\"}],\"packageUris\":[\"http://schema.mathworks.com/mf0/Connector/R2020b\"],\"version\":\"1.0\"}"
  S1 : Outport
  S2 : Outport  Port=2
  S3 : Outport  Port=3
  S4 : Outport  Port=4
  wires:
  ? -> S1/1
  ? -> S2/1
  ? -> S3/1
  ? -> S4/1
  V1/1 -> Balancing chart/4(v1)
  V2/1 -> Balancing chart/2(v2)
  V3/1 -> Balancing chart/3(v3)
  V4/1 -> Balancing chart/1(v4)

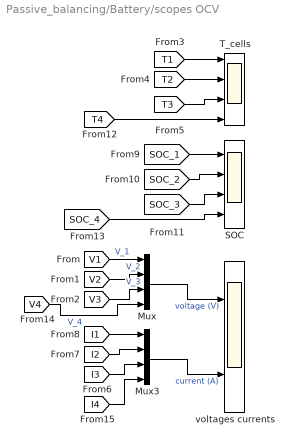
== system Passive_balancing/Battery/scopes OCV ==
  Mux : Mux
  Mux3 : Mux
  SOC : Scope  NumInputPorts=4
  T_cells : Scope  NumInputPorts=4
  voltages currents : Scope  NumInputPorts=2
  wires:
  [I3] -> Mux3/3
  [V1] -> Mux/1  "V_1"
  [V3] -> Mux/3  "V_3"
  Mux/1 -> voltages currents/1  "voltage (V)"
  [V2] -> Mux/2  "V_2"
  [I1] -> Mux3/1
  [I2] -> Mux3/2
  Mux3/1 -> voltages currents/2  "current (A)"
  [SOC_1] -> SOC/1
  [SOC_2] -> SOC/2
  [SOC_3] -> SOC/3
  [T1] -> T_cells/1
  [T2] -> T_cells/2
  [T3] -> T_cells/3
  [T4] -> T_cells/4
  [SOC_4] -> SOC/4
  [V4] -> Mux/4  "V_4"
  [I4] -> Mux3/4

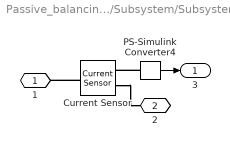
== system Passive_balancing/Battery/Subsystem/Subsystem1 ==
  Current Sensor : fl_lib/Electrical/Electrical Sensors/Current Sensor
  PS-Simulink Converter4 : nesl_utility/PS-Simulink Converter  PhysicalDomain=network_engine_domain  SubClassName=ps_output  LeftPortType=input  RightPortType=output  PseudoPeriodic=off  Frequencies=[]  Unit=1  AffineConversion=off
  1 : PMIOPort  Side=Left
  2 : PMIOPort  Port=2  Side=Right
  3 : Outport  VectorParamsAs1DForOutWhenUnconnected=off
  wires:
  PS-Simulink Converter4/1 -> 3/1
  connections:
  PS-Simulink Converter4/LConn1 -- Current Sensor/RConn1
  Current Sensor/RConn2 -- 2/RConn1
  Current Sensor/LConn1 -- 1/RConn1

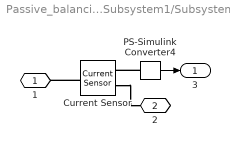
== system Passive_balancing/Battery/Subsystem1/Subsystem2 ==
  Current Sensor : fl_lib/Electrical/Electrical Sensors/Current Sensor
  PS-Simulink Converter4 : nesl_utility/PS-Simulink Converter  PhysicalDomain=network_engine_domain  SubClassName=ps_output  LeftPortType=input  RightPortType=output  PseudoPeriodic=off  Frequencies=[]  Unit=1  AffineConversion=off
  1 : PMIOPort  Side=Left
  2 : PMIOPort  Port=2  Side=Right
  3 : Outport  VectorParamsAs1DForOutWhenUnconnected=off
  wires:
  PS-Simulink Converter4/1 -> 3/1
  connections:
  PS-Simulink Converter4/LConn1 -- Current Sensor/RConn1
  Current Sensor/RConn2 -- 2/RConn1
  Current Sensor/LConn1 -- 1/RConn1

== system Passive_balancing/Battery/Subsystem3/Subsystem ==
  Current Sensor : fl_lib/Electrical/Electrical Sensors/Current Sensor
  PS-Simulink Converter4 : nesl_utility/PS-Simulink Converter  PhysicalDomain=network_engine_domain  SubClassName=ps_output  LeftPortType=input  RightPortType=output  PseudoPeriodic=off  Frequencies=[]  Unit=1  AffineConversion=off
  1 : PMIOPort  Side=Left
  2 : PMIOPort  Port=2  Side=Right
  3 : Outport  VectorParamsAs1DForOutWhenUnconnected=off
  wires:
  PS-Simulink Converter4/1 -> 3/1
  connections:
  Current Sensor/LConn1 -- 1/RConn1
  Current Sensor/RConn2 -- 2/RConn1
  PS-Simulink Converter4/LConn1 -- Current Sensor/RConn1

== system Passive_balancing/Battery/Subsystem6/Subsystem2 ==
  Current Sensor : fl_lib/Electrical/Electrical Sensors/Current Sensor
  PS-Simulink Converter4 : nesl_utility/PS-Simulink Converter  PhysicalDomain=network_engine_domain  SubClassName=ps_output  LeftPortType=input  RightPortType=output  PseudoPeriodic=off  Frequencies=[]  Unit=1  AffineConversion=off
  1 : PMIOPort  Side=Left
  2 : PMIOPort  Port=2  Side=Right
  3 : Outport  VectorParamsAs1DForOutWhenUnconnected=off
  wires:
  PS-Simulink Converter4/1 -> 3/1
  connections:
  PS-Simulink Converter4/LConn1 -- Current Sensor/RConn1
  Current Sensor/RConn2 -- 2/RConn1
  Current Sensor/LConn1 -- 1/RConn1

== stateflow chart Passive_balancing/Chart ==
  state wait
  state DISCH
    du: MODE = 2;
  state CH
    du: MODE = 1;
  (default) -> wait
  wait -> (junction 14)
  (junction 14) -> (junction 16) [order 1] : [SOC_MAX<0.5]
  (junction 14) -> DISCH [order 2] : [SOC_MAX>=0.5]
  (junction 16) -> (junction 19)
  CH -> DISCH : [SOC_MAX > 0.99 || after(5000,sec)]
  DISCH -> CH : [SOC_min < 0.3]
  (junction 19) -> CH
  data: MODE output; SOC_MAX input; SOC_min input

== stateflow chart Passive_balancing/Battery/Subsystem8/Balancing chart ==
  state finish
    entry: s1 = 0;
    s2 = 0;
    s3 = 0;
    s4=0;
  state init
    entry: s1 = 0;
    s2 = 0;
    s3 = 0;
    s4 = 0;
  state balancing
    du: sortV = ord(v1,v2,v3,v4);
    state s4_s1_s2
      en: s2 = 1;
      s3 = 0;
      s4=1;
      s2=1
      ex: s1 = 0;
      s3 = 0;
      s2 = 0;
      s4=0;
    state s1_s2_s3
      en: s1 = 1;
      s3=1;
      s2 = 1;
      s4 = 0;
      ex: s1 = 0;
      s2 = 0;
      s3 = 0;
      s4=0;
    state s3_s4_s1
      en: s1 = 1;
      s3 = 1;
      s4=1;
      s2 = 0;
      ex: s1 = 0;
      s3 = 0;
      s2 = 0;
      s4=0;
    state s2_s3_s4
      en: s1 = 0;
      s2 = 1;
      s3 = 1;
      s4=1;
      ex: s1 = 0;
      s2 = 0;
      s3 = 0;
      s4=0;
    (default) -> (junction 38) : {sortV = ord(v1,v2,v3,v4);}
    (junction 38) -> s1_s2_s3 [order 3] : [sortV(1)==4]
    (junction 38) -> (junction 39) [order 2] : % cell#1 lowest
        | [sortV(1)==3]
    (junction 38) -> (junction 1) [order 1] : % cell#2 lowest
        | [sortV(1)==2]
    (junction 38) -> (junction 55) [order 4]
    (junction 39) -> s4_s1_s2
    (junction 1) -> (junction 2)
    (junction 55) -> s2_s3_s4
    (junction 2) -> s3_s4_s1
    s2_s3_s4 -> s3_s4_s1 [order 1] : [sortV(1)==2]
    s3_s4_s1 -> s4_s1_s2 [order 2] : [sortV(1)==3]
    s2_s3_s4 -> s1_s2_s3 [order 2] : [sortV(1)==4]
    s3_s4_s1 -> s2_s3_s4 [order 1] : [sortV(1)==1]
    s4_s1_s2 -> s3_s4_s1 [order 1] : [sortV(1)==2]
    s1_s2_s3 -> s2_s3_s4 [order 1] : [sortV(1)==1]
    s4_s1_s2 -> (junction 3) [order 2] : [sortV(1)==4]
    (junction 4) -> s4_s1_s2
    (junction 42) -> s1_s2_s3
    s1_s2_s3 -> (junction 48) [order 2]
    (junction 3) -> (junction 42)
    (junction 48) -> (junction 4) : [sortV(1)==3]
  (default) -> init
  finish -> balancing : [abs(max([v1 v2 v3 v4]) - min([v1 v2 v3 v4])) > deltaV && after(1,sec)]
  balancing -> finish : [abs(max([v1 v2 v3 v4]) - min([v1 v2 v3 v4])) < deltaV]
  init -> balancing : [abs(max([v1 v2 v3 v4]) - min([v1 v2 v3 v4])) > deltaV]
  data: a function_input; b function_input; c function_input; p function_output; d function_input; v4 input; v2 input; v3 input; v1 input; sortV parameter; s1 output; s4 output; s3 output; s2 output
  function p = ord(a,b,c,d):
    | function p = ord(a,b,c,d)
    | [~,p] = sort([a,b,c,d],'ascend');
